simulink model "procsenales2_ej1"  (Simulink 7.3)
settings: Solver=ode45  StartTime=0.0  StopTime=200.0  RelTol=1e-3
values from neighbouring files (symbols this model uses):
  h = tiempo(2)-tiempo(1)    [a290916_sesgo.m]    (also in p06092016.m = 1; p20092016_TI.m = 1; p20092016_sesgo.m = 1)
libraries: simulink x1
settings Model: Creator=alumno  LastModifiedBy=alumno

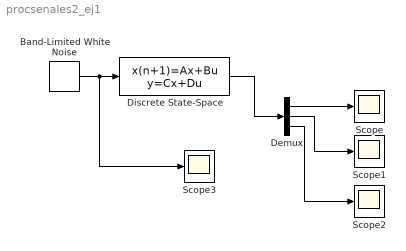
== system procsenales2_ej1 ==
  Band-Limited White Noise : simulink/Sources/Band-Limited White Noise  SystemSampleTime=-1  Cov=[0.001 0.002 0.004]'  Ts=h  seed=[rand()*1000 rand()*1000 rand()*1000]
  Demux : Demux  Outputs=3
  Discrete State-Space : DiscreteStateSpace  A=[1 h 0.5*h^2;0 1 h;0 0 1]  B=eye(3)  C=eye(3)  D=zeros(3)  SampleTime=h
  Scope{,1..3} (4 alike) : Scope
      Scope2 settings: SaveName=ScopeData2
      Scope3 settings: SaveName=ScopeData3
  wires:
  Band-Limited White Noise/1 -> Discrete State-Space/1, Scope3/1
  Discrete State-Space/1 -> Demux/1
  Demux/1 -> Scope/1
  Demux/2 -> Scope1/1
  Demux/3 -> Scope2/1
